simulink model "Task3FSK"  (R2024a)
settings: Solver=VariableStepAuto  StartTime=0.0  StopTime=30  RelTol=1e-3
libraries: commrandsrc3 x1
settings Model: Creator=17760  LastModifiedBy=17760

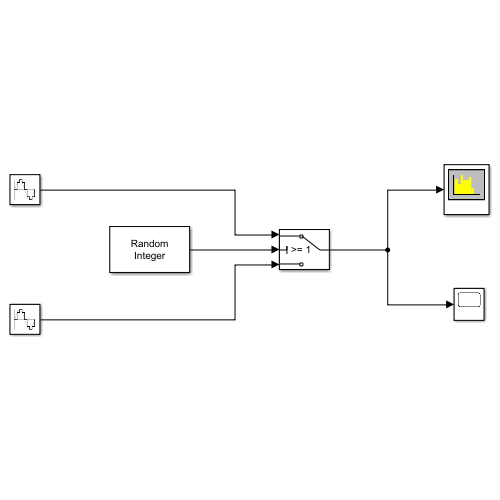
[thumbnail: Simulink's stored preview of the top-level diagram]
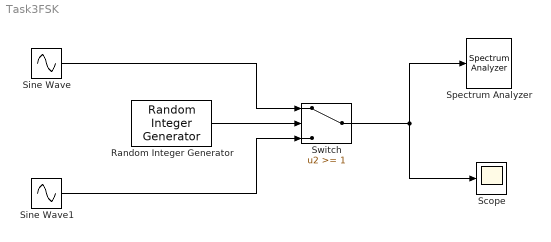
== system Task3FSK ==
  Random Integer Generator : commrandsrc3/Random Integer Generator  SetSize=2  SeedSource=Auto  Seed=0  SampleTime=1  SamplesPerFrame=1  OutputDataType=single  SimulateUsing=Code generation
  Scope : Scope
  Sine Wave : Sin  Frequency=2*pi*10  SampleTime=1/100
  Sine Wave1 : Sin  Frequency=2*pi*5  SampleTime=1/100
  Spectrum Analyzer : SpectrumAnalyzer  WindowPosition=[1.000000,49.000000,1440.000000,889.000000,]  ScopeFrameLocation=window  YLimits=[-1.6397800459793972,0.9907178895138156]
  Switch : Switch  Threshold=1  SaturateOnIntegerOverflow=off  InputSameDT=off
  wires:
  Random Integer Generator/1 -> Switch/2
  Sine Wave/1 -> Switch/1
  Switch/1 -> Scope/1, Spectrum Analyzer/1
  Sine Wave1/1 -> Switch/3
